simulink model "ver_sim2"  (Simulink 8.9)
settings: Solver=ode15s  StartTime=0.0  StopTime=10.0  RelTol=1e-3
values from neighbouring files (symbols this model uses):
  b = 0.01    [K_Gain_matrix.m]    (also in Lab2.m = B; Stepper_Model_2017_10_31_Script.m; Stepper_Model_2017_Mark_Script.m)
  M = 1.2    [K_Gain_matrix.m]    (also in Lab2.m = P(1); Stepper_Model_2017_10_31_Script.m; Stepper_Model_2017_Mark_Script.m)
settings Model: Creator=c3204612  LastModifiedBy=Administrator
settings DataIOCC: LimitDataPoints=off  SaveFormat=Dataset  SignalLoggingSaveFormat=Dataset
settings DebuggingCC: UnderspecifiedInitializationDetection=Simplified  MergeDetectMultiDrivingBlocksExec=error  FcnCallInpInsideContextMsg=error  StateNameClashWarn=none  SFUnexpectedBacktrackingDiag=error  SFNoUnconditionalDefaultTransitionDiag=error
settings HardwareCC: ProdBitPerPointer=64  ProdBitPerSizeT=64  ProdBitPerPtrDiffT=64  ProdLargestAtomicFloat=Float  ProdIntDivRoundTo=Zero  ProdEndianess=LittleEndian  ProdWordSize=64  ProdHWDeviceType=Intel->x86-64 (Windows64)
settings ModelReferenceCC: PropagateSignalLabelsOutOfModel=on
settings GRTTargetCC: TargetLangStandard=C99 (ISO)  GeneratePreprocessorConditionals=Use local settings  CombineOutputUpdateFcns=on  GRTInterface=off
settings ConfigComp: CovMetricSettings=dwe  CovHtmlReporting=off  CovSaveCumulativeToWorkspaceVar=off  CovSaveSingleToWorkspaceVar=off  CovExternalEMLEnable=on

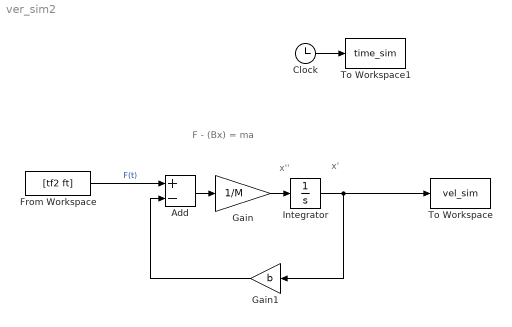
== system ver_sim2 ==
  note: F - (Bx) = ma
  note: x'
  note: x''
  Add : Sum  Inputs=+-
  Clock : Clock
  From Workspace : FromWorkspace  VariableName=[tf2 ft]  SampleTime=0
  Gain : Gain  Gain=1/M
  Gain1 : Gain  Gain=b
  Integrator : Integrator
  To Workspace : ToWorkspace  VariableName=vel_sim  SampleTime=-1
  To Workspace1 : ToWorkspace  VariableName=time_sim  SampleTime=-1
  wires:
  From Workspace/1 -> Add/1  "F(t)"
  Add/1 -> Gain/1
  Gain/1 -> Integrator/1
  Integrator/1 -> To Workspace/1, Gain1/1
  Gain1/1 -> Add/2
  Clock/1 -> To Workspace1/1
